simulink model "bh_smd_COMP_MASKED_MDL"  (R2018a)
settings: Solver=ode4  StartTime=0.0  StopTime=10.0  FixedStep=0.01  RelTol=1e-7
model mask{m=1, c=2*0.5*5, k=25, x_init=0, xdot_init=0}
  mask prompts: m "What is the m:"; c "What is the c:"; k "What is the k:"; x_init "Initial Position"; xdot_init "Initial Velocity"
model workspace (MAT data in the model file):
  c = 2.5
  k = 25
  m = 1
  x_init = 5
  xdot_init = 0
settings Model: ParameterArgumentNames=c,k,m,x_init,xdot_init  OrderedModelArguments=off  Creator=bhorton  LastModifiedBy=bhorton
settings CodeAppCC: StateflowObjectComments=on

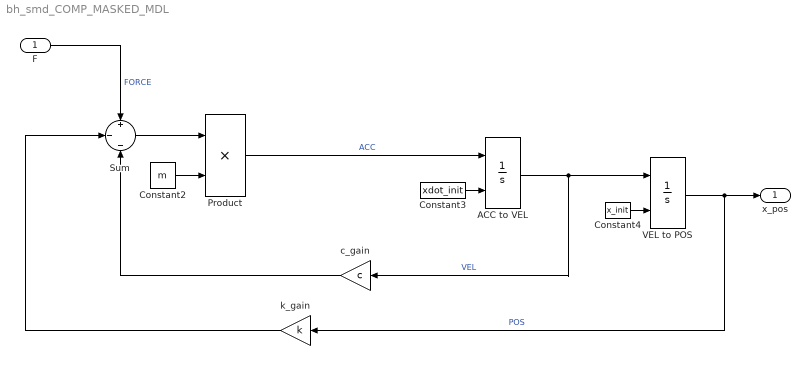
== system bh_smd_COMP_MASKED_MDL ==
  F : Inport
  ACC to VEL : Integrator  InitialConditionSource=external
  Constant2 : Constant  Value=m
  Constant3 : Constant  Value=xdot_init
  Constant4 : Constant  Value=x_init
  Product : Product
  Sum : Sum  Inputs=+|-|-
  VEL to POS : Integrator  InitialConditionSource=external
  c_gain : Gain  Gain=c
  k_gain : Gain  Gain=k
  x_pos : Outport
  wires:
  F/1 -> Sum/1  "FORCE"
  Product/1 -> ACC to VEL/1  "ACC"
  ACC to VEL/1 -> c_gain/1, VEL to POS/1  "VEL"
  VEL to POS/1 -> x_pos/1, k_gain/1  "POS"
  Constant2/1 -> Product/2
  Constant3/1 -> ACC to VEL/2
  Constant4/1 -> VEL to POS/2
  Sum/1 -> Product/1
  c_gain/1 -> Sum/3
  k_gain/1 -> Sum/2
